simulink model "balance_car_with_fuzzy_logic"  (R2023b)
settings: Solver=VariableStepAuto  StartTime=0.0  StopTime=80  RelTol=1e-3
values from neighbouring files (symbols this model uses):
  d = 0.1612    [new_parameter.m]    (also in parameter.m)
  g = 9.8    [new_parameter.m]    (also in parameter.m)
  I = 0.5*m*r^2    (= 1.3475e-05)    [new_parameter.m]    (also in parameter.m = 1.97568e-05)
  J_delta = (1/12)*M*(0.0930^2+0.0530^2)    (= 0.000680796166667)    [new_parameter.m]    (also in parameter.m = 0.0006559705)
  J_p = (1/12)*M*(0.3^2+0.08^2)    (= 0.00572776666667)    [new_parameter.m]    (also in parameter.m = 0.0006276369025)
  l = 0.5*0.8    (= 0.4)    [new_parameter.m]    (also in parameter.m = 0.04515)
  M = 0.757-2*m    (= 0.713)    [new_parameter.m]    (also in parameter.m = 0.687)
  m = 0.022    [new_parameter.m]    (also in parameter.m = 0.035)
  r = 0.07/2    (= 0.035)    [new_parameter.m]    (also in parameter.m = 0.0336)
  Ts = 0.1    [new_parameter.m]    (also in parameter.m)
libraries: simulink x3, fuzblock x2, slpidlib x1
settings Model: Creator=zhy  LastModifiedBy=zhy

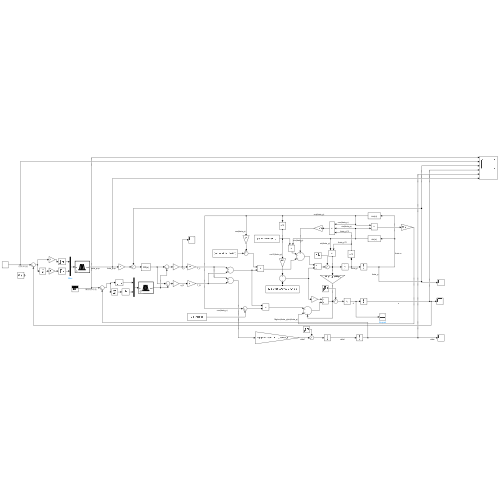
[thumbnail: Simulink's stored preview of the top-level diagram]
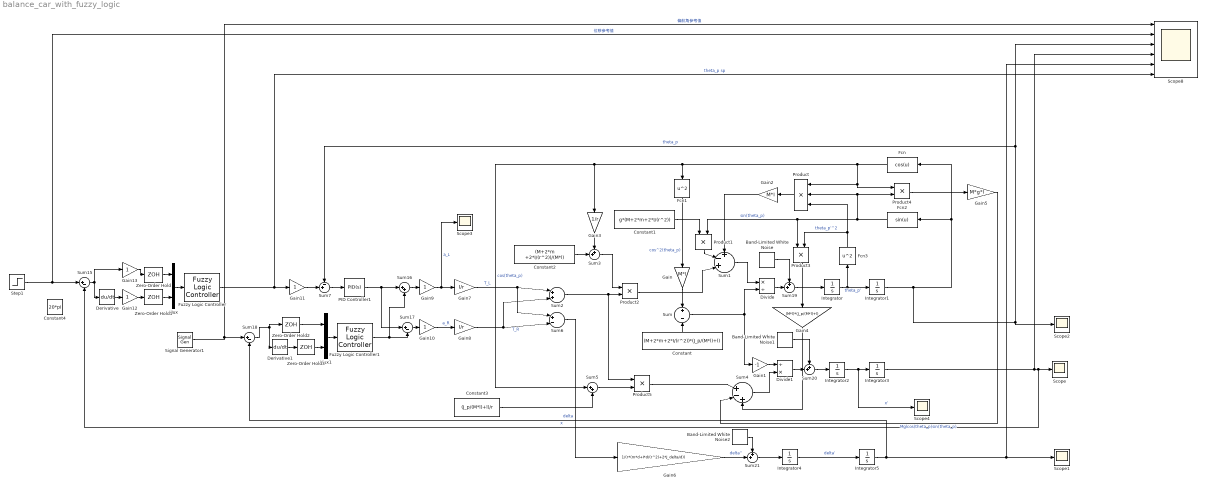
== system balance_car_with_fuzzy_logic ==
  Band-Limited White Noise : simulink/Sources/Band-Limited White Noise  Cov=[0.0001]  Ts=0.1  seed=[23341]
  Band-Limited White Noise1 : simulink/Sources/Band-Limited White Noise  Cov=[0.0001]  Ts=0.1  seed=[23342]
  Band-Limited White Noise2 : simulink/Sources/Band-Limited White Noise  Cov=[0.001]  Ts=0.1  seed=[23343]
  Constant : Constant  Value=(M+2*m+2*I/(r^2))*(J_p/(M*l)+l)
  Constant1 : Constant  Value=g*(M+2*m+2*I/(r^2))
  Constant2 : Constant  Value=(M+2*m +2*I/(r^2))/(M*l)
  Constant3 : Constant  Value=(J_p/(M*l)+l)/r
  Constant4 : Constant  Value=20*pi
  Derivative : Derivative
  Derivative1 : Derivative
  Divide : Product  Inputs=*/
  Divide1 : Product  Inputs=/*
  Fcn : Fcn  Expr=cos(u)
  Fcn1 : Fcn  Expr=u^2
  Fcn2 : Fcn  Expr=sin(u)
  Fcn3 : Fcn  Expr=u^2
  Fuzzy Logic Controller : fuzblock/Fuzzy Logic  Controller  FIS='fuzzy_controller.fis'  OutputSampleNumber=101  DataType=double  FuzzifiedInputs=off  RuleFiringStrengths=off  RuleOutputs=off  AggregatedOutputs=off  SimulateUsing=Interpreted execution  OutOfRangeInputValueMessage=warning  NoRuleFiredMessage=warning  EmptyOutputFuzzySetMessage=warning
  Fuzzy Logic Controller1 : fuzblock/Fuzzy Logic  Controller  FIS='fuzzy_delta.fis'  OutputSampleNumber=101  DataType=double  FuzzifiedInputs=off  RuleFiringStrengths=off  RuleOutputs=off  AggregatedOutputs=off  SimulateUsing=Interpreted execution  OutOfRangeInputValueMessage=warning  NoRuleFiredMessage=warning  EmptyOutputFuzzySetMessage=warning
  Gain : Gain  Gain=M*l
  Gain1 : Gain  Gain=-1
  Gain{9..13} (5 alike) : Gain
  Gain2 : Gain  Gain=M*l
  Gain3 : Gain  Gain=1/r
  Gain4 : Gain  Gain=(M*l)*(J_p/(M*l)+l)
  Gain5 : Gain  Gain=M*g*l
  Gain6 : Gain  Gain=1/(r*(m*d+I*d/(r^2)+2*J_delta/d))
  Gain7 : Gain  Gain=I/r
  Gain8 : Gain  Gain=I/r
  Integrator{,1..5} (6 alike) : Integrator
  Mux : Mux  Inputs=2
  Mux1 : Mux  Inputs=2
  PID Controller1 : slpidlib/PID Controller  Controller=PID  Form=Parallel  TimeDomain=Continuous-time  UseExternalTs=off  SampleTime=-1  IntegratorMethod=Forward Euler  FilterMethod=Forward Euler  ControllerParametersSource=internal  P=-280  I=-200  UseKiTs=off  D=-120  N=100000  UseFilter=on  TunerSelectOption=Transfer Function Based (PID Tuner App)  InitialConditionSource=internal  InitialConditionForIntegrator=0  InitialConditionForFilter=0  DifferentiatorICPrevScaledInput=0  ExternalReset=none  TrackingMode=off  Kt=1  LimitOutput=off  SatLimitsSource=internal  UpperSaturationLimit=inf  LowerSaturationLimit=-inf  LinearizeAsGain=on  AntiWindupMode=none  Kb=1  LimitIntegrator=off  UpperIntegratorSaturationLimit=inf  LowerIntegratorSaturationLimit=-inf  POutMin=[]  POutMax=[]  IOutMin=[]  IOutMax=[]  DOutMin=[]  DOutMax=[]  NOutMin=[]  NOutMax=[]  SumOutMin=[]  SumOutMax=[]  SaturationOutMin=[]  SaturationOutMax=[]  PParamMin=[]  PParamMax=[]  IParamMin=[]  IParamMax=[]  DParamMin=[]  DParamMax=[]  NParamMin=[]  NParamMax=[]  KbParamMin=[]  KbParamMax=[]  KtParamMin=[]  KtParamMax=[]  KbOutMin=[]  KbOutMax=[]  KtOutMin=[]  KtOutMax=[]  IntegratorOutMin=[]  IntegratorOutMax=[]  FilterOutMin=[]  FilterOutMax=[]  SumI1OutMin=[]  SumI1OutMax=[]  SumI2OutMin=[]  SumI2OutMax=[]  SumI3OutMin=[]  SumI3OutMax=[]  SumI4OutMin=[]  SumI4OutMax=[]  SumDOutMin=[]  SumDOutMax=[]  DifferentiatorOutMin=[]  DifferentiatorOutMax=[]  FilterDiffOutCoefMin=[]  FilterDiffOutCoefMax=[]  ReciprocalOutMin=[]  ReciprocalOutMax=[]  SumDenOutMin=[]  SumDenOutMax=[]  SumNumOutMin=[]  SumNumOutMax=[]  DivideOutMin=[]  DivideOutMax=[]  UdiffTsProdOutMin=[]  UdiffTsProdOutMax=[]  NTsProdOutMin=[]  NTsProdOutMax=[]  UintegralTsProdOutMin=[]  UintegralTsProdOutMax=[]  UngainTsProdOutMin=[]  UngainTsProdOutMax=[]  ClampingZeroOutDataTypeStr=Inherit: Inherit via back propagation  ClampingZeroOutMin=[]  ClampingZeroOutMax=[]  FilterDenConstantOutDataTypeStr=Inherit: Inherit via back propagation  FilterDenConstantOutMin=[]  FilterDenConstantOutMax=[]  PCopyOutDataTypeStr=Inherit: Inherit via back propagation  PCopyOutMin=[]  PCopyOutMax=[]  NCopyOutDataTypeStr=Inherit: Inherit via back propagation  NCopyOutMin=[]  NCopyOutMax=[]  IntegratorContinuousStateAttributes=''  IntegratorStateMustResolveToSignalObject=off  IntegratorRTWStateStorageClass=Auto  FilterContinuousStateAttributes=''  FilterStateMustResolveToSignalObject=off  FilterRTWStateStorageClass=Auto  ParallelPVariant=InternalParameters  IdealPVariant=Disabled  IVariant=InternalParameters  DVariant=InternalParameters  IntegratorVariant=Continuous  SatVariant=Disabled  AWVariant=Passthrough  PCopyVariant=Disabled  TRVariant=Disabled  FdbkBlocksVariant=Forward  IdealPFdbkVariant=Disabled  SatFdbkVariant=Disabled  DerivativeFilterVariant=ContFilter  NVariant=InternalParameters  NCopyVariant=Disabled  FilterICVariant=InternalICsFilter  IntegratorICVariant=InternalICs  ExternalResetVariant=Disabled  TRSumVariant=Passthrough  SumFdbkVariant=Disabled  SumVariant=Sum_PID  TsampFilterVariant=InternalTs  TsampNgainVariant=Passthrough  TsampIntegralVariant=Disabled_SignalSpec  ExternalSaturationOutDataTypeStr=Inherit: Same as second input
  Product : Product  Inputs=3
  Product{1..5} (5 alike) : Product
  Scope{,1..4} (5 alike) : Scope
  Scope8 : Scope  NumInputPorts=6
  Signal Generator1 : SignalGenerator  Amplitude=0.1  Frequency=0.05
  Step1 : Step  Time=5  After=0.5  SampleTime=0
  Sum : Sum  Inputs=+-
  Sum1 : Sum  Inputs=+-+|
  Sum15 : Sum  Inputs=|+-
  Sum16 : Sum  Inputs=|++
  Sum17 : Sum  Inputs=|+-
  Sum18 : Sum  Inputs=|+-
  Sum{3,19..21} (4 alike) : Sum  Inputs=++|
  Sum2 : Sum  Inputs=|++|
  Sum4 : Sum  Inputs=|+-+
  Sum5 : Sum  Inputs=|++
  Sum6 : Sum  Inputs=|+-|
  Sum7 : Sum  Inputs=-+|
  Zero-Order Hold{,1..3} (4 alike) : ZeroOrderHold  SampleTime=Ts
  wires:
  Product5/1 -> Sum4/1
  Sum19/1 -> Integrator/1
  Fcn/1 -> Product4/1, Product/1, Fcn1/1, Sum5/1, Gain3/1  "cos(theta_p)"
  Sum17/1 -> Gain10/1
  Fcn2/1 -> Product1/2, Product3/1, Product4/2, Product/2  "sin(theta_p)"
  Sum1/1 -> Divide/1
  Sum7/1 -> PID Controller1/1
  Sum3/1 -> Product2/1
  Gain9/1 -> Scope3/1, Gain7/1  "a_L"
  Gain8/1 -> Sum6/2, Sum2/2  "T_R"
  Divide/1 -> Sum19/2
  Integrator1/1 -> Scope8/3, Sum7/1, Scope2/1, Fcn2/1, Fcn/1  "theta_p"
  Fcn1/1 -> Gain/1  "cos^2(theta_p)"
  Gain2/1 -> Sum1/1
  Gain10/1 -> Gain8/1  "a_R"
  Gain4/1 -> Sum4/3
  Product3/1 -> Gain4/1
  Sum5/1 -> Product5/2
  Constant2/1 -> Sum3/2
  Product4/1 -> Gain5/1
  Gain7/1 -> Sum6/1, Sum2/1  "T_L"
  PID Controller1/1 -> Sum16/1, Sum17/1
  Sum6/1 -> Gain6/1
  Integrator2/1 -> Scope4/1, Integrator3/1  "x'"
  Sum/1 -> Gain1/1, Divide/2
  Integrator3/1 -> Scope/1, Sum15/2, Scope8/4  "x"
  Constant/1 -> Sum/2
  Constant1/1 -> Product1/1
  Sum2/1 -> Product5/1, Product2/2
  Fcn3/1 -> Product/3, Product3/2  "theta_p'^2"
  Product1/1 -> Sum1/2
  Gain3/1 -> Sum3/1
  Constant3/1 -> Sum5/2
  Gain5/1 -> Sum4/2  "Mglcos(theta_p)sin(theta_p)"
  Product2/1 -> Sum1/3
  Gain/1 -> Sum/1
  Integrator4/1 -> Integrator5/1  "delta'"
  Band-Limited White Noise1/1 -> Sum20/1
  Integrator/1 -> Integrator1/1, Fcn3/1  "theta_p'"
  Signal Generator1/1 -> Sum18/1, Scope8/1  "偏航角参考值"
  Sum16/1 -> Gain9/1
  Product/1 -> Gain2/1
  Band-Limited White Noise/1 -> Sum19/1
  Sum21/1 -> Integrator4/1
  Sum20/1 -> Integrator2/1
  Gain1/1 -> Divide1/1
  Step1/1 -> Sum15/1, Scope8/2  "位移参考值"
  Gain6/1 -> Sum21/2  "delta''"
  Integrator5/1 -> Scope8/5, Scope1/1, Sum18/2  "delta"
  Sum4/1 -> Divide1/2
  Divide1/1 -> Sum20/2
  Band-Limited White Noise2/1 -> Sum21/1
  Gain11/1 -> Sum7/2
  Gain12/1 -> Zero-Order Hold1/1
  Mux/1 -> Fuzzy Logic Controller/1
  Fuzzy Logic Controller/1 -> Scope8/6, Gain11/1  "theta_p sp"
  Sum15/1 -> Derivative/1, Gain13/1
  Gain13/1 -> Zero-Order Hold/1
  Zero-Order Hold/1 -> Mux/1
  Zero-Order Hold1/1 -> Mux/2
  Derivative/1 -> Gain12/1
  Zero-Order Hold3/1 -> Mux1/2
  Zero-Order Hold2/1 -> Mux1/1
  Derivative1/1 -> Zero-Order Hold3/1
  Mux1/1 -> Fuzzy Logic Controller1/1
  Sum18/1 -> Zero-Order Hold2/1, Derivative1/1
  Fuzzy Logic Controller1/1 -> Sum17/2, Sum16/2
